simulink model "PD_Controller_RBF_SupervisoryControl_2021b"  (R2021b)
settings: Solver=FixedStepDiscrete  StartTime=0.0  StopTime=0.2  FixedStep=0.0001  RelTol=1e-3
values from neighbouring files (symbols this model uses):
  kd = 13.4    [phy_param_RBF_Control.m]
  kp = 44.5    [phy_param_RBF_Control.m]
undefined symbols (not defined in the file or in its folder): den, num
libraries: simulink x2
settings Model: Creator=auw_a  LastModifiedBy=auw_a
settings DebuggingCC: UnconnectedInputMsg=none  UnconnectedOutputMsg=none  UnconnectedLineMsg=none
settings ModelReferenceCC: EnableRefExpFcnMdlSchedulingChecks=off
settings RTWCC: DLArmComputeVersion=20.02.1

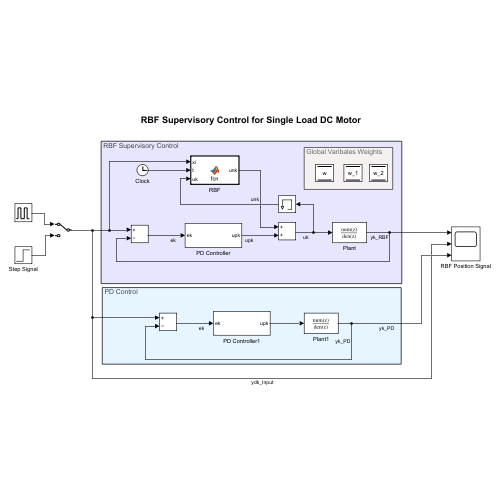
[thumbnail: Simulink's stored preview of the top-level diagram]
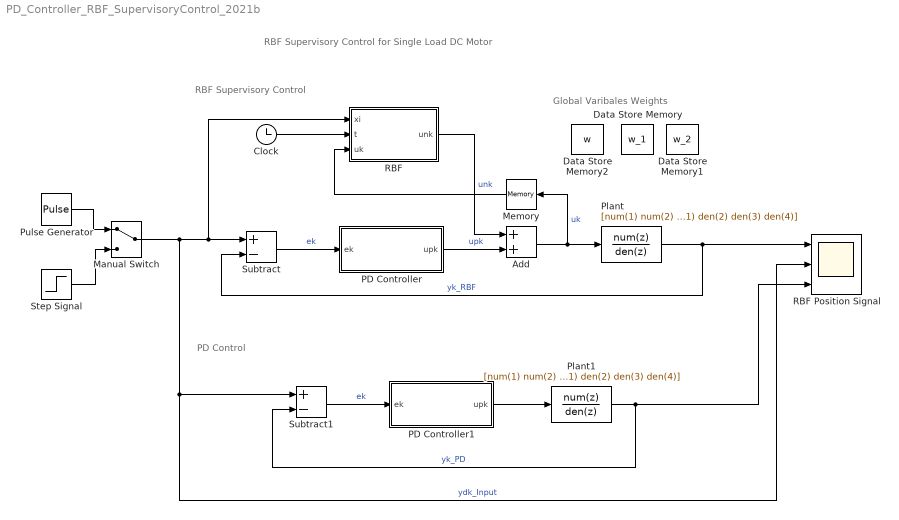
== system PD_Controller_RBF_SupervisoryControl_2021b ==
  note: PD Control
  note: Global Varibales Weights
  note: RBF Supervisory Control for Single Load DC Motor
  note: RBF Supervisory Control
  Add : Sum
  Clock : Clock
  Data Store Memory : DataStoreMemory  DataStoreName=w_1  WriteAfterWriteMsg=warning  InitialValue=[0; 0; 0; 0]  ShowAdditionalParam=off  OutDataTypeStr=double
  Data Store Memory1 : DataStoreMemory  DataStoreName=w_2  WriteAfterWriteMsg=warning  InitialValue=[0; 0; 0; 0]  ShowAdditionalParam=off  OutDataTypeStr=double
  Data Store Memory2 : DataStoreMemory  DataStoreName=w  WriteAfterWriteMsg=warning  InitialValue=[0; 0; 0; 0]  ShowAdditionalParam=off  OutDataTypeStr=double
  Manual Switch : ManualSwitch
  Memory : Memory
  PD Controller : Subsystem
  PD Controller1 : Subsystem
  Plant : DiscreteTransferFcn  Numerator=[num(1) num(2) num(3) num(4)]  Denominator=[den(1) den(2) den(3) den(4)]
  Plant1 : DiscreteTransferFcn  Numerator=[num(1) num(2) num(3) num(4)]  Denominator=[den(1) den(2) den(3) den(4)]
  Pulse Generator : DiscretePulseGenerator  PulseType=Time based  Period=0.4  PulseWidth=50
  RBF : MATLAB Function  TreatAsAtomicUnit=on
  RBF Position Signal : Scope  NumInputPorts=3
  Step Signal : Step  Time=0  SampleTime=0.0001
  Subtract : Sum  Inputs=+-
  Subtract1 : Sum  Inputs=+-
  wires:
  Plant/1 -> Subtract/2, RBF Position Signal/1  "yk_RBF"
  Subtract/1 -> PD Controller/1(ek)  "ek"
  RBF/1(unk) -> Add/1  "unk"
  PD Controller/1(upk) -> Add/2  "upk"
  Add/1 -> Memory/1, Plant/1  "uk"
  Clock/1 -> RBF/2(t)
  Memory/1 -> RBF/3(uk)
  PD Controller1/1(upk) -> Plant1/1
  Subtract1/1 -> PD Controller1/1(ek)  "ek"
  Step Signal/1 -> Manual Switch/2
  Plant1/1 -> Subtract1/2, RBF Position Signal/3  "yk_PD"
  Manual Switch/1 -> Subtract1/1, RBF Position Signal/2, RBF/1(xi), Subtract/1  "ydk_Input"
  Pulse Generator/1 -> Manual Switch/1

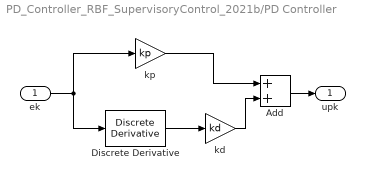
== system PD_Controller_RBF_SupervisoryControl_2021b/PD Controller ==
  ek : Inport
  Add : Sum
  Discrete Derivative : simulink/Discrete/Discrete Derivative  gainval=1.0  ICPrevScaledInput=0.0  OutMin=[]  OutMax=[]  OutDataType=fixdt(1, 16)  OutScaling=2^-10  DoSatur=off
  kd : Gain  Gain=kd
  kp : Gain  Gain=kp
  upk : Outport
  wires:
  Discrete Derivative/1 -> kd/1
  kp/1 -> Add/1
  kd/1 -> Add/2
  Add/1 -> upk/1
  ek/1 -> Discrete Derivative/1, kp/1

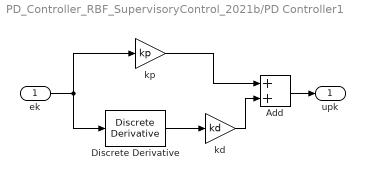
== system PD_Controller_RBF_SupervisoryControl_2021b/PD Controller1 ==
  ek : Inport
  Add : Sum
  Discrete Derivative : simulink/Discrete/Discrete Derivative  gainval=1.0  ICPrevScaledInput=0.0  OutMin=[]  OutMax=[]  OutDataType=fixdt(1, 16)  OutScaling=2^-10  DoSatur=off
  kd : Gain  Gain=kd
  kp : Gain  Gain=kp
  upk : Outport
  wires:
  ek/1 -> kp/1, Discrete Derivative/1
  Add/1 -> upk/1
  kd/1 -> Add/2
  kp/1 -> Add/1
  Discrete Derivative/1 -> kd/1

== matlab function PD_Controller_RBF_SupervisoryControl_2021b/RBF ==
  data: unk output; xi input; t input; uk input; w data_store_memory; w_1 data_store_memory; w_2 data_store_memory
function unk = fcn(xi, t, uk)

global w w_1 w_2

% initializing global variables
if isempty(w)
    w = zeros(4,1);
end
if isempty(w_1)
    w_1 = zeros(4,1);
end
if isempty(w_2)
    w_2 = zeros(4,1);
end

xite = 0.30;            % learning rate
alfa = 0.05;            % momentum factor

b = 0.5*ones(4,1);    % vector b - width of Gaussian Function
c = [-4 -2 2 4];      % coordinate valve of center point of Gaussian Function

if t == 0
    uk = 0;
    w = rand(4,1);        % weight vector of RBF
    w_1 = w;
    w_2 = w_1;
end

h = zeros(1, 4);        % Gaussian Function vector
% calculating RB vector
for a=1:1:4
    h(a) = exp(-norm(xi-c(:,a))^2/(2*b(a)*b(a)));
end

unk = (w' * h');      % output of the RBF

%Update NN Weight
d_w = -xite*(unk-uk)*(h');
w_temp = w_1 + d_w + alfa*(w_1 - w_2);
w = w_temp;
w_2 = w_1;
w_1 = w;
